simulink model "totalSystem"  (R2019b)
settings: Solver=FixedStepAuto  StartTime=0.0  StopTime=100.0  FixedStep=0.001  RelTol=1e-3
values from neighbouring files (symbols this model uses):
  ballLQRgain = lqr(ballSystem, Q, R)    [init.m]
  ballPosInit = [0.1;0;0;0]    [init.m]
  C_v = 16.5    [init.m]
  g = 9.81    [init.m]
  I0 = (m_p+3*m_m)*g/(3*K)    (= 0.37278)    [init.m]
  I_b = m_b*r_b^2    (= 8.664e-06)    [init.m]
  I_p = m_p*0.04^2/12    (= 0.00012)    [init.m]
  K = 11    [init.m]
  m_b = 0.024    [init.m]
  m_m = 0.118    [init.m]
  m_p = 0.9    [init.m]
  motorPlateInit = [0;0;0;0;0;0.32]    [init.m]
  r = 0.17    [init.m]
  r_b = 0.019    [init.m]
undefined symbols (not defined in the file or in its folder): Continuous, denc_mi, numc_mi, Time
libraries: ctrlSharedLib x1
settings Model: Creator=chukh  LastModifiedBy=chukh

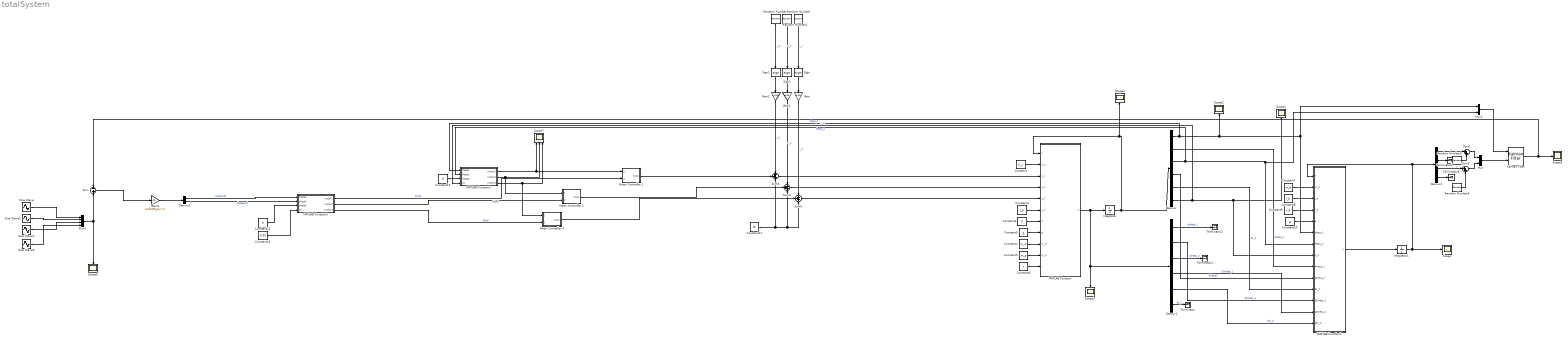
== system totalSystem ==
  Constant : Constant  Value=C_v
  Constant1 : Constant  Value=I_p
  Constant10 : Constant  Value=g
  Constant11 : Constant  Value=I0
  Constant12 : Constant  Value=0
  Constant13 : Constant  Value=0
  Constant14 : Constant  Value=0.32
  Constant2 : Constant  Value=K
  Constant3 : Constant  Value=g
  Constant4 : Constant  Value=m_m
  Constant5 : Constant  Value=m_p
  Constant6 : Constant  Value=r
  Constant7 : Constant  Value=m_b
  Constant8 : Constant  Value=I_b
  Constant9 : Constant  Value=r_b
  Demux : Demux  Outputs=6
  Demux1 : Demux  Outputs=6
  Demux2 : Demux
  Demux3 : Demux  Outputs=2
  Gain : Gain  Gain=0.05
  Gain1 : Gain  Gain=0.05
  Gain2 : Gain  Gain=0.05
  Gain3 : Gain  Gain=ballLQRgain  Multiplication=Matrix(K*u)
  Integrator : Integrator  InitialCondition=motorPlateInit
  Integrator1 : Integrator  InitialCondition=ballPosInit
  Kalman Filter : ctrlSharedLib/Kalman Filter  TimeDomain=Continuous-Time  UseCurrentEstimator=on  ModelSource=LTI State-Space Variable  ModelSourceVariable=ballSystem  A=0.95  B=1  C=1  D=0  NumberOfStates=1  NumberOfInputs=1  NumberOfOutputs=1  InitialEstimateSource=Dialog  X0=ballPosInit  P0=10  UseK=off  UseGH=off  NumberOfProcessNoiseInputs=1  G=1  TimeInvariantG=on  H=0  TimeInvariantH=on  Q=0.05  TimeInvariantQ=on  R=1  TimeInvariantR=on  N=0  TimeInvariantN=on  AddInputPort=on  AddEnablePort=off  OutputEstimatedY=off  OutputP=off  Ts=-1
      settings: SourceProductBaseCode=CT
  MATLAB Function : MATLAB Function  TreatAsAtomicUnit=on
  MATLAB Function1 : MATLAB Function  TreatAsAtomicUnit=on
  MATLAB Function2 : MATLAB Function  TreatAsAtomicUnit=on
  MATLAB Function3 : MATLAB Function  TreatAsAtomicUnit=on
  Motor Controller 1 : Subsystem
  Motor Controller 2 : Subsystem
  Motor Controller 3 : Subsystem
  Mux : Mux  Inputs=2
  Mux1 : Mux  Inputs=2
  Mux2 : Mux
  Random Number : RandomNumber  Seed=13  SampleTime=0.001
  Random Number1 : RandomNumber  Seed=23  SampleTime=0.001
  Random Number2 : RandomNumber  Seed=47  SampleTime=0.001
  Random Number3 : RandomNumber  Variance=0.005  Seed=193  SampleTime=0
  Random Number4 : RandomNumber  Variance=0.005  Seed=98676  SampleTime=0
  Scope{,1..6} (7 alike) : Scope
  Scope7 : Scope  NumInputPorts=3
  Sign : Signum
  Sign1 : Signum
  Sign2 : Signum
  Sine Wave : Sin  Amplitude=0.1  Frequency=pi/5  Phase=pi/2  SampleTime=0
  Sine Wave1 : Sin  Amplitude=0.1  Frequency=pi/5  SampleTime=0
  Sine Wave2 : Sin  Amplitude=0.1  Phase=pi  SampleTime=0
  Sine Wave3 : Sin  Amplitude=0.1  Phase=pi/2  SampleTime=0
  Sum : Sum  Inputs=-+
  Sum1 : Sum  Inputs=|++
  Sum2 : Sum  Inputs=|++
  Sum3 : Sum  Inputs=+++
  Sum4 : Sum  Inputs=+++
  Sum5 : Sum  Inputs=+++
  Terminator{,1..4} (5 alike) : Terminator
  wires:
  Demux/6 -> Scope1/1, MATLAB Function1/8(z_C), MATLAB Function2/4(Zc)  "z_C"
  Demux/2 -> MATLAB Function1/9(dtheta_1)  "dtheta_1"
  Demux/3 -> Mux1/2, MATLAB Function1/7(theta_2), MATLAB Function2/2(theta2)  "theta_2"
  Demux/4 -> MATLAB Function1/10(dtheta_2)  "dtheta2"
  Demux/5 -> MATLAB Function1/11(dz_C)  "dz_C"
  Demux1/6 -> Terminator/1  "dz_C"
  Demux1/1 -> Terminator2/1  "dtheta_1"
  Demux1/2 -> MATLAB Function1/12(d2theta_1)  "d2theta_1"
  Demux1/3 -> Terminator1/1  "dtheta_2"
  Demux1/4 -> MATLAB Function1/13(d2theta_2)  "d2theta_2"
  Demux1/5 -> MATLAB Function1/14(d2z_C)  "d2z_C"
  MATLAB Function1/1(V) -> Integrator1/1
  Integrator1/1 -> Scope/1, MATLAB Function1/1(Y), Demux2/1
  Constant7/1 -> MATLAB Function1/2(m_b)
  Constant8/1 -> MATLAB Function1/3(I_b)
  Constant9/1 -> MATLAB Function1/4(r_b)
  Constant10/1 -> MATLAB Function1/5(g)
  Demux/1 -> Scope2/1, MATLAB Function1/6(theta_1), Mux1/1, MATLAB Function2/1(theta1)  "theta_1"
  Constant5/1 -> MATLAB Function/10(m_p)
  MATLAB Function/1(V) -> Demux1/1, Scope3/1, Integrator/1
  Random Number/1 -> Sign/1  "I_1"
  Constant4/1 -> MATLAB Function/9(m_m)
  Integrator/1 -> Demux/1, Scope4/1, MATLAB Function/1(Y)
  Constant/1 -> MATLAB Function/2(C_v)
  Constant2/1 -> MATLAB Function/7(K)
  Random Number2/1 -> Sign2/1  "I_3"
  Constant6/1 -> MATLAB Function/11(r)
  Constant1/1 -> MATLAB Function/6(I_p)
  Random Number1/1 -> Sign1/1  "I_2"
  Constant3/1 -> MATLAB Function/8(g)
  Sign/1 -> Gain/1
  Sign1/1 -> Gain1/1
  Sign2/1 -> Gain2/1
  Sum3/1 -> MATLAB Function/4(I_2)
  Gain1/1 -> Sum3/1  "I_2"
  Gain2/1 -> Sum4/1  "I_1"
  Sum5/1 -> MATLAB Function/5(I_3)
  Constant11/1 -> Sum3/3, Sum5/3, Sum4/3
  Gain/1 -> Sum5/1  "I_3"
  Sum4/1 -> MATLAB Function/3(I_1)
  Constant12/1 -> MATLAB Function2/3(theta3)
  MATLAB Function2/1(motor1) -> Scope7/1, Motor Controller 1/1(Output)
  MATLAB Function3/1(motor1) -> Motor Controller 1/2(Reference)  "P1ref"
  Motor Controller 1/1(Out1) -> Sum4/2
  MATLAB Function3/2(motor2) -> Motor Controller 2/2(Reference)  "P2ref"
  MATLAB Function3/3(motor3) -> Motor Controller 3/2(Reference)  "P3ref"
  MATLAB Function2/2(motor2) -> Scope7/2, Motor Controller 2/1(Output)
  MATLAB Function2/3(motor3) -> Scope7/3, Motor Controller 3/1(Output)
  Motor Controller 3/1(Out1) -> Sum5/2
  Motor Controller 2/1(Out1) -> Sum3/2
  Demux2/2 -> Terminator3/1
  Demux2/4 -> Terminator4/1
  Demux2/1 -> Sum1/1  "x"
  Demux2/3 -> Sum2/1  "y"
  Mux/1 -> Kalman Filter/2
  Mux1/1 -> Kalman Filter/1
  Kalman Filter/1 -> Sum/1, Scope5/1
  Demux3/1 -> MATLAB Function3/1(theta1)  "theta1ref"
  Demux3/2 -> MATLAB Function3/2(theta2)  "theta2ref"
  Constant13/1 -> MATLAB Function3/3(theta3)
  Constant14/1 -> MATLAB Function3/4(Zc)
  Gain3/1 -> Demux3/1
  Sum/1 -> Gain3/1
  Sine Wave1/1 -> Mux2/3
  Mux2/1 -> Scope6/1, Sum/2
  Sine Wave2/1 -> Mux2/2
  Sine Wave/1 -> Mux2/1
  Sine Wave3/1 -> Mux2/4
  Random Number3/1 -> Sum1/2
  Random Number4/1 -> Sum2/2
  Sum2/1 -> Mux/2
  Sum1/1 -> Mux/1

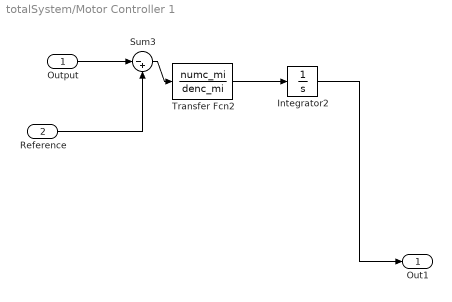
== system totalSystem/Motor Controller 1 ==
  Output : Inport
  Reference : Inport  Port=2
  Integrator2 : Integrator
  Sum3 : Sum  Inputs=|-+
  Transfer Fcn2 : TransferFcn  Numerator=numc_mi  Denominator=denc_mi
  Out1 : Outport
  wires:
  Transfer Fcn2/1 -> Integrator2/1
  Sum3/1 -> Transfer Fcn2/1
  Output/1 -> Sum3/1
  Reference/1 -> Sum3/2
  Integrator2/1 -> Out1/1

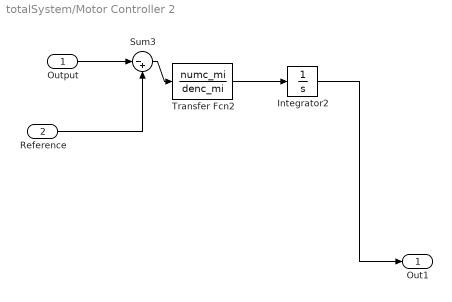
== system totalSystem/Motor Controller 2 ==
  Output : Inport
  Reference : Inport  Port=2
  Integrator2 : Integrator
  Sum3 : Sum  Inputs=|-+
  Transfer Fcn2 : TransferFcn  Numerator=numc_mi  Denominator=denc_mi
  Out1 : Outport
  wires:
  Transfer Fcn2/1 -> Integrator2/1
  Sum3/1 -> Transfer Fcn2/1
  Output/1 -> Sum3/1
  Reference/1 -> Sum3/2
  Integrator2/1 -> Out1/1

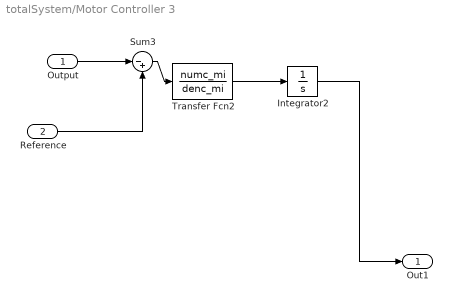
== system totalSystem/Motor Controller 3 ==
  Output : Inport
  Reference : Inport  Port=2
  Integrator2 : Integrator
  Sum3 : Sum  Inputs=|-+
  Transfer Fcn2 : TransferFcn  Numerator=numc_mi  Denominator=denc_mi
  Out1 : Outport
  wires:
  Transfer Fcn2/1 -> Integrator2/1
  Sum3/1 -> Transfer Fcn2/1
  Output/1 -> Sum3/1
  Reference/1 -> Sum3/2
  Integrator2/1 -> Out1/1

== matlab function totalSystem/MATLAB Function1 ==
  data: Y input; V output; m_b input; I_b input; r_b input; g input; theta_1 input; theta_2 input; z_C input; dtheta_1 input; dtheta_2 input; dz_C input; d2theta_1 input; d2theta_2 input; d2z_C input
function V = ballOnPlateODE(Y,m_b,I_b,r_b,g,theta_1,theta_2,z_C,dtheta_1,dtheta_2,dz_C,d2theta_1,d2theta_2,d2z_C)
%BALLONPLATEODE
%    V = BALLONPLATEODE(Y,M_B,I_B,R_B,G,THETA_1,THETA_2,Z_C,DTHETA_1,DTHETA_2,DZ_C,D2THETA_1,D2THETA_2,D2Z_C)

%    This function was generated by the Symbolic Math Toolbox version 8.4.
%    16-May-2021 00:03:52

%matrix([[xf], [Dxf], [yf], [Dyf]])
t2 = cos(theta_1);
t3 = cos(theta_2);
t4 = sin(theta_1);
t5 = sin(theta_2);
t6 = Y(1);
t7 = Y(2);
t8 = Y(3);
t9 = Y(4);
t10 = dtheta_1.^2;
t11 = dtheta_2.^2;
t12 = r_b.^2;
t13 = r_b.^3;
t14 = t2.^2;
t15 = t2.^3;
t16 = t3.^2;
t18 = t3.^3;
t20 = t4.^2;
t21 = t4.^3;
t22 = t5.^2;
t24 = t5.^3;
t28 = m_b.*t12;
t17 = t14.^2;
t19 = t16.^2;
t23 = t20.^2;
t25 = t22.^2;
t26 = 1.0./t14;
t27 = 1.0./t16;
t29 = I_b+t28;
t30 = t14+t20;
t31 = 1.0./t29;
t32 = 1.0./t30;
V = [t7;(t26.*t27.*t31.*t32.*(I_b.*d2theta_2.*r_b.*t15.*t18+I_b.*r_b.*t11.*t15.*t24.*2.0-I_b.*t6.*t11.*t17.*t19-I_b.*t6.*t11.*t17.*t25.*2.0+d2z_C.*t5.*t17.*t18.*t28+g.*t5.*t17.*t18.*t28+m_b.*t11.*t13.*t15.*t24.*2.0-t6.*t11.*t17.*t25.*t28.*2.0+d2theta_2.*m_b.*t3.*t13.*t15.*t22+d2theta_1.*t5.*t8.*t16.*t17.*t28-d2theta_2.*t5.*t6.*t17.*t18.*t28-d2theta_2.*t3.*t6.*t17.*t24.*t28+dtheta_1.*t5.*t9.*t16.*t17.*t28.*2.0-dtheta_2.*t5.*t7.*t17.*t18.*t28.*2.0+dtheta_1.*t5.*t9.*t17.*t18.*t28-dtheta_2.*t3.*t7.*t17.*t24.*t28.*2.0+m_b.*t5.*t10.*t13.*t15.*t16.*2.0+m_b.*t5.*t11.*t13.*t15.*t16+t4.*t8.*t11.*t15.*t24.*t28.*2.0-t6.*t10.*t16.*t17.*t22.*t28-t6.*t11.*t16.*t17.*t22.*t28.*2.0+I_b.*dtheta_1.*dtheta_2.*r_b.*t18.*t21.*2.0+I_b.*dtheta_1.*dtheta_2.*t8.*t17.*t18.*2.0-I_b.*dtheta_1.*dtheta_2.*t8.*t17.*t19+I_b.*dtheta_1.*dtheta_2.*t8.*t18.*t23.*2.0+I_b.*d2theta_2.*r_b.*t2.*t18.*t20+I_b.*d2theta_2.*r_b.*t3.*t15.*t22+I_b.*d2theta_1.*t5.*t8.*t16.*t17+I_b.*d2theta_2.*t4.*t8.*t15.*t18-I_b.*d2theta_2.*t5.*t6.*t17.*t18-I_b.*d2theta_1.*t5.*t8.*t17.*t18+I_b.*d2theta_2.*t2.*t8.*t18.*t21-I_b.*d2theta_2.*t3.*t6.*t17.*t24+I_b.*dtheta_1.*t5.*t9.*t16.*t17.*2.0+I_b.*dtheta_2.*t4.*t9.*t15.*t18.*2.0-I_b.*dtheta_2.*t5.*t7.*t17.*t18.*2.0-I_b.*dtheta_1.*t5.*t9.*t17.*t18+I_b.*dtheta_2.*t2.*t9.*t18.*t21.*2.0-I_b.*dtheta_2.*t3.*t7.*t17.*t24.*2.0+I_b.*r_b.*t5.*t10.*t15.*t16+I_b.*r_b.*t5.*t11.*t15.*t16.*2.0+I_b.*r_b.*t2.*t11.*t20.*t24.*2.0+I_b.*t4.*t8.*t11.*t15.*t24.*2.0+I_b.*t2.*t8.*t11.*t21.*t24.*2.0-I_b.*t6.*t11.*t14.*t19.*t20-I_b.*t6.*t11.*t16.*t17.*t22.*3.0-I_b.*t6.*t11.*t14.*t20.*t25.*2.0+I_b.*dtheta_1.*dtheta_2.*r_b.*t4.*t14.*t18.*2.0-I_b.*dtheta_1.*dtheta_2.*r_b.*t4.*t14.*t22+I_b.*dtheta_1.*dtheta_2.*r_b.*t3.*t21.*t22.*2.0+I_b.*dtheta_1.*dtheta_2.*t4.*t6.*t15.*t24+I_b.*dtheta_1.*dtheta_2.*t3.*t8.*t17.*t22.*2.0+I_b.*dtheta_1.*dtheta_2.*t3.*t8.*t22.*t23.*2.0+I_b.*dtheta_1.*dtheta_2.*t8.*t14.*t18.*t20.*4.0-I_b.*dtheta_1.*dtheta_2.*t8.*t14.*t19.*t20-I_b.*dtheta_1.*dtheta_2.*t8.*t14.*t20.*t22-I_b.*d2theta_1.*r_b.*t3.*t4.*t5.*t14+I_b.*d2theta_1.*r_b.*t4.*t5.*t14.*t16+I_b.*d2theta_2.*r_b.*t2.*t3.*t20.*t22+I_b.*d2theta_1.*t3.*t4.*t6.*t15.*t22-I_b.*d2theta_1.*t3.*t5.*t8.*t14.*t20+I_b.*d2theta_2.*t3.*t4.*t8.*t15.*t22+I_b.*d2theta_2.*t2.*t3.*t8.*t21.*t22+I_b.*d2theta_1.*t5.*t8.*t14.*t16.*t20-I_b.*d2theta_2.*t5.*t6.*t14.*t18.*t20-I_b.*d2theta_2.*t3.*t6.*t14.*t20.*t24+I_b.*dtheta_1.*t3.*t4.*t7.*t15.*t22-I_b.*dtheta_1.*t3.*t5.*t9.*t14.*t20+I_b.*dtheta_2.*t3.*t4.*t9.*t15.*t22.*2.0+I_b.*dtheta_2.*t2.*t3.*t9.*t21.*t22.*2.0+I_b.*dtheta_1.*t5.*t9.*t14.*t16.*t20.*2.0-I_b.*dtheta_2.*t5.*t7.*t14.*t18.*t20.*2.0-I_b.*dtheta_2.*t3.*t7.*t14.*t20.*t24.*2.0+I_b.*r_b.*t2.*t5.*t10.*t16.*t20+I_b.*r_b.*t2.*t5.*t11.*t16.*t20.*2.0-I_b.*t3.*t4.*t5.*t8.*t10.*t15+I_b.*t4.*t5.*t8.*t10.*t15.*t16+I_b.*t4.*t5.*t8.*t11.*t15.*t16.*2.0+I_b.*t4.*t5.*t8.*t10.*t15.*t18+I_b.*t2.*t5.*t8.*t10.*t16.*t21+I_b.*t2.*t5.*t8.*t11.*t16.*t21.*2.0-I_b.*t3.*t6.*t10.*t14.*t20.*t22-I_b.*t6.*t11.*t14.*t16.*t20.*t22.*3.0+dtheta_1.*dtheta_2.*m_b.*t4.*t13.*t14.*t22-dtheta_1.*dtheta_2.*t4.*t6.*t15.*t24.*t28+dtheta_1.*dtheta_2.*t3.*t8.*t17.*t22.*t28.*2.0+dtheta_1.*dtheta_2.*t8.*t14.*t20.*t22.*t28+d2theta_1.*m_b.*t4.*t5.*t13.*t14.*t16+d2theta_2.*t3.*t4.*t8.*t15.*t22.*t28+d2theta_1.*t5.*t8.*t14.*t16.*t20.*t28-dtheta_1.*t3.*t4.*t7.*t15.*t22.*t28+dtheta_1.*t3.*t5.*t9.*t14.*t20.*t28+dtheta_2.*t3.*t4.*t9.*t15.*t22.*t28.*2.0+dtheta_1.*t5.*t9.*t14.*t16.*t20.*t28.*2.0+m_b.*t2.*t3.*t5.*t10.*t13.*t20.*2.0+m_b.*t2.*t5.*t10.*t13.*t16.*t20+t3.*t4.*t5.*t8.*t10.*t15.*t28+t2.*t3.*t5.*t8.*t10.*t21.*t28.*2.0+t4.*t5.*t8.*t10.*t15.*t16.*t28+t4.*t5.*t8.*t11.*t15.*t16.*t28+t4.*t5.*t8.*t10.*t15.*t18.*t28+t2.*t5.*t8.*t10.*t16.*t21.*t28-t3.*t6.*t10.*t14.*t20.*t22.*t28+I_b.*dtheta_1.*dtheta_2.*r_b.*t3.*t4.*t14.*t22.*2.0+I_b.*dtheta_1.*dtheta_2.*t4.*t5.*t6.*t15.*t16+I_b.*dtheta_1.*dtheta_2.*t3.*t8.*t14.*t20.*t22.*4.0-I_b.*dtheta_1.*dtheta_2.*t8.*t14.*t16.*t20.*t22+dtheta_1.*dtheta_2.*m_b.*t3.*t4.*t13.*t14.*t22.*2.0+dtheta_1.*dtheta_2.*t3.*t8.*t14.*t20.*t22.*t28.*2.0))./(t16+t22);t9;-t26.*t27.*t31.*t32.*(I_b.*d2theta_1.*r_b.*t3.*t15+I_b.*r_b.*t10.*t16.*t21.*2.0+I_b.*t3.*t8.*t10.*t17+I_b.*t8.*t10.*t16.*t17-I_b.*t8.*t10.*t17.*t18+I_b.*t8.*t10.*t16.*t23.*2.0+d2z_C.*t4.*t15.*t18.*t28+g.*t4.*t15.*t18.*t28+m_b.*t10.*t13.*t16.*t21.*2.0-t3.*t8.*t10.*t17.*t28+t8.*t10.*t16.*t17.*t28.*2.0-t8.*t10.*t17.*t18.*t28+t8.*t10.*t16.*t23.*t28.*2.0+d2theta_1.*m_b.*t2.*t13.*t16.*t20+d2theta_1.*t4.*t8.*t15.*t16.*t28-d2theta_2.*t4.*t6.*t15.*t18.*t28+d2theta_1.*t2.*t8.*t16.*t21.*t28-dtheta_1.*t3.*t4.*t9.*t15.*t28+dtheta_1.*t3.*t5.*t7.*t17.*t28+dtheta_1.*t4.*t9.*t15.*t16.*t28.*2.0-dtheta_2.*t4.*t7.*t15.*t18.*t28.*2.0+dtheta_1.*t4.*t9.*t15.*t18.*t28+dtheta_1.*t2.*t9.*t16.*t21.*t28.*2.0-m_b.*t3.*t4.*t10.*t13.*t14.*2.0+m_b.*t4.*t10.*t13.*t14.*t16.*3.0+m_b.*t4.*t11.*t13.*t14.*t16+m_b.*t4.*t11.*t13.*t14.*t22.*2.0-t3.*t8.*t10.*t14.*t20.*t28.*2.0-t4.*t6.*t11.*t15.*t24.*t28.*2.0+t8.*t10.*t14.*t16.*t20.*t28.*4.0+t8.*t11.*t14.*t16.*t20.*t28+t8.*t11.*t14.*t20.*t22.*t28.*2.0+I_b.*dtheta_1.*dtheta_2.*r_b.*t5.*t15-I_b.*dtheta_1.*dtheta_2.*t6.*t16.*t17-I_b.*dtheta_1.*dtheta_2.*t6.*t17.*t22+I_b.*d2theta_1.*r_b.*t2.*t16.*t20+I_b.*d2theta_1.*t3.*t4.*t8.*t15-I_b.*d2theta_1.*t3.*t5.*t6.*t17+I_b.*d2theta_1.*t4.*t8.*t15.*t16-I_b.*d2theta_1.*t4.*t8.*t15.*t18+I_b.*d2theta_1.*t2.*t8.*t16.*t21+I_b.*dtheta_1.*t3.*t4.*t9.*t15-I_b.*dtheta_1.*t3.*t5.*t7.*t17+I_b.*dtheta_1.*t4.*t9.*t15.*t16.*2.0-I_b.*dtheta_1.*t4.*t9.*t15.*t18+I_b.*dtheta_1.*t2.*t9.*t16.*t21.*2.0+I_b.*r_b.*t4.*t10.*t14.*t16.*2.0+I_b.*t8.*t10.*t14.*t16.*t20.*3.0-dtheta_1.*dtheta_2.*m_b.*t5.*t13.*t15+dtheta_1.*dtheta_2.*t6.*t17.*t22.*t28+I_b.*dtheta_1.*dtheta_2.*t4.*t5.*t8.*t15+I_b.*t3.*t4.*t5.*t6.*t10.*t15-dtheta_1.*dtheta_2.*t4.*t5.*t8.*t15.*t28+d2theta_2.*m_b.*t3.*t4.*t5.*t13.*t14-d2theta_2.*t3.*t4.*t6.*t15.*t22.*t28+d2theta_2.*t3.*t5.*t8.*t14.*t20.*t28-dtheta_2.*t3.*t4.*t7.*t15.*t22.*t28.*2.0+dtheta_2.*t3.*t5.*t9.*t14.*t20.*t28.*2.0+t3.*t4.*t5.*t6.*t10.*t15.*t28-t4.*t5.*t6.*t10.*t15.*t16.*t28-t4.*t5.*t6.*t11.*t15.*t16.*t28.*2.0+I_b.*dtheta_1.*dtheta_2.*t4.*t5.*t8.*t15.*t16+dtheta_1.*dtheta_2.*m_b.*t2.*t3.*t5.*t13.*t20.*2.0+dtheta_1.*dtheta_2.*t3.*t4.*t5.*t8.*t15.*t28.*2.0+dtheta_1.*dtheta_2.*t2.*t3.*t5.*t8.*t21.*t28.*2.0)];

== matlab function totalSystem/MATLAB Function ==
  data: V output; Y input; C_v input; I_1 input; I_2 input; I_3 input; I_p input; K input; g input; m_m input; m_p input; r input
function V = motorPlateODE(Y,C_v,I_1,I_2,I_3,I_p,K,g,m_m,m_p,r)
%MOTORPLATEODE
%    V = MOTORPLATEODE(T,Y,C_V,I_1,I_2,I_3,I_P,K,G,M_M,M_P,R)

%    This function was generated by the Symbolic Math Toolbox version 8.4.
%    18-May-2021 19:45:09

%matrix([[theta_1f], [omega_1f], [theta_2f], [omega_2f], [dz_Cf], [z_Cf]])
t2 = I_p.^2;
t3 = Y(1);
t4 = Y(2);
t5 = Y(3);
t6 = Y(4);
t7 = Y(5);
t8 = m_m.^2;
t9 = r.^2;
t10 = r.^3;
t19 = sqrt(3.0);
t11 = t9.^2;
t12 = cos(t3);
t13 = cos(t5);
t14 = sin(t3);
t15 = sin(t5);
t16 = t2.*4.0;
t17 = t4.^2;
t18 = t6.^2;
t20 = t12.^2;
t21 = t12.^3;
t22 = t13.^2;
t23 = t13.^3;
t25 = t14.^2;
t26 = t15.^2;
t24 = t22.^2;
t27 = I_p.*m_m.*t9.*t22.*6.0;
t29 = I_p.*m_m.*t9.*t25.*t26.*6.0;
t28 = t20.*t27;
t30 = t8.*t11.*t20.*t24.*9.0;
t31 = t16+t27+t28+t29+t30;
t32 = 1.0./t31;
V = [t4;t32.*(t12.*t14.*t17.*t27+t12.*t14.*t18.*t27+t8.*t11.*t12.*t14.*t17.*t24.*9.0+t8.*t11.*t12.*t14.*t18.*t24.*9.0-C_v.*I_p.*t4.*t9.*t20.*t22.*6.0-C_v.*m_m.*t4.*t11.*t20.*t24.*9.0+I_2.*I_p.*K.*r.*t12.*t13.*t19.*2.0-I_3.*I_p.*K.*r.*t12.*t13.*t19.*2.0+I_2.*K.*m_m.*t10.*t12.*t19.*t23.*3.0-I_3.*K.*m_m.*t10.*t12.*t19.*t23.*3.0+t4.*t6.*t8.*t11.*t15.*t20.*t23.*1.8e+1+t8.*t11.*t12.*t14.*t18.*t22.*t26.*1.8e+1-t8.*t11.*t14.*t18.*t21.*t22.*t26.*9.0-t8.*t11.*t12.*t14.^3.*t18.*t22.*t26.*9.0-t4.*t6.*t8.*t11.*t13.*t15.^3.*t20.*t25.*9.0+C_v.*I_p.*t6.*t9.*t12.*t13.*t14.*t15.*6.0-I_1.*K.*m_m.*t10.*t12.*t14.*t15.*t22.*6.0+I_2.*K.*m_m.*t10.*t12.*t14.*t15.*t22.*3.0+I_3.*K.*m_m.*t10.*t12.*t14.*t15.*t22.*3.0+I_p.*m_m.*t4.*t6.*t9.*t13.*t15.*t20.*1.2e+1+t4.*t6.*t8.*t11.*t13.*t15.*t20.*t25.*9.0-t4.*t6.*t8.*t11.*t15.*t20.*t23.*t25.*9.0);t6;-r.*t32.*(I_1.*I_p.*K.*t13.*4.0-I_2.*I_p.*K.*t13.*2.0-I_3.*I_p.*K.*t13.*2.0+C_v.*I_p.*r.*t6.*t22.*6.0-t8.*t10.*t15.*t18.*t20.*t23.*1.8e+1+t8.*t10.*t15.*t18.*t20.^2.*t23.*9.0+I_2.*I_p.*K.*t14.*t15.*t19.*2.0-I_3.*I_p.*K.*t14.*t15.*t19.*2.0+C_v.*I_p.*r.*t6.*t25.*t26.*6.0+I_1.*K.*m_m.*t9.*t20.*t23.*6.0-I_2.*K.*m_m.*t9.*t20.*t23.*3.0-I_3.*K.*m_m.*t9.*t20.*t23.*3.0+C_v.*m_m.*t6.*t10.*t20.*t24.*9.0-I_p.*m_m.*r.*t13.*t15.*t18.*1.2e+1-I_p.*m_m.*r.*t4.*t6.*t12.*t14.*6.0+I_p.*m_m.*r.*t13.*t15.*t18.*t20.*6.0+I_p.*m_m.*r.*t13.*t15.*t17.*t25.*6.0+I_p.*m_m.*r.*t13.*t15.*t18.*t25.*1.2e+1-t4.*t6.*t8.*t10.*t14.*t21.*t22.*9.0+t4.*t6.*t8.*t10.*t14.*t21.*t24.*9.0+t8.*t10.*t15.*t18.*t20.*t23.*t25.*9.0-C_v.*I_p.*r.*t4.*t12.*t13.*t14.*t15.*6.0+I_p.*m_m.*r.*t4.*t6.*t12.*t14.*t22.*6.0+I_p.*m_m.*r.*t4.*t6.*t12.*t14.*t26.*1.8e+1+t4.*t6.*t8.*t10.*t14.*t21.*t22.*t26.*9.0);-(C_v.*t7.*3.0+g.*m_m.*3.0+g.*m_p-I_1.*K-I_2.*K-I_3.*K)./(m_m.*3.0+m_p);t7];

== matlab function totalSystem/MATLAB Function2 ==
  data: theta1 input; motor1 output; theta2 input; theta3 input; Zc input; motor2 output; motor3 output
% Roll-Pitch-Yaw angles to motors position
% Roll (theta1): rotation about x-axis
% Pitch (theta2): rotation about y-axis
% Yaw (theta3): rotation about z-axis
% See page 12 and Appendix A (Multibody and Nonlinear Dynamics lecture
% notes for further reference
% Motors (1,2,3) -> (A,B,C)

function [motor1, motor2, motor3] = anglesToMotors(theta1,theta2,theta3,Zc)

%% Define parameters
r = 0.17;
r0B1 = [r; 0; 0];      
r0B2 = [-0.5*r; (sqrt(3)/2)*r; 0];
r0B3 = [-0.5*r; -(sqrt(3)/2)*r; 0];
r0B = [r0B1 r0B2 r0B3];
%r1C1 = r0B1; r1C2 = r0B2; r1C3 = r0B3;
r1C = r0B;
r0Oc = [0;0;Zc];

% Find cos and sin to accelerate calculations
C1 = cos(theta1);S1 = sin(theta1);C2 = cos(theta2);S2 = sin(theta2);C3 = cos(theta3);S3 = sin(theta3);

% Rotation matrices
RotZ = [C3 S3 0; -S3 C3 0; 0 0 1];
RotY = [C2 0 -S2; 0 1 0; S2 0 C2];
RotX = [1 0 0; 0 C1 S1; 0 -S1 C1];

A10 = RotX*RotY*RotZ; A01 = A10';

% Find rCiBi (Vectors representing the motors)
rCiBi = zeros(3,3);
for i=1:3
    rCiBi(:,i) = r0Oc + A01*r1C(:,i) - r0B(:,i);
end

% Outputs to motor are the lengths of the vectors
motor1 = norm(rCiBi(:,1));
motor2 = norm(rCiBi(:,2));
motor3 = norm(rCiBi(:,3));
end

== matlab function totalSystem/MATLAB Function3 ==
  data: theta1 input; motor1 output; theta2 input; theta3 input; Zc input; motor2 output; motor3 output
% Roll-Pitch-Yaw angles to motors position
% Roll (theta1): rotation about x-axis
% Pitch (theta2): rotation about y-axis
% Yaw (theta3): rotation about z-axis
% See page 12 and Appendix A (Multibody and Nonlinear Dynamics lecture
% notes for further reference
% Motors (1,2,3) -> (A,B,C)

function [motor1, motor2, motor3] = anglesToMotors(theta1,theta2,theta3,Zc)

%% Define parameters
r = 0.17;
r0B1 = [r; 0; 0];      
r0B2 = [-0.5*r; (sqrt(3)/2)*r; 0];
r0B3 = [-0.5*r; -(sqrt(3)/2)*r; 0];
r0B = [r0B1 r0B2 r0B3];
%r1C1 = r0B1; r1C2 = r0B2; r1C3 = r0B3;
r1C = r0B;
r0Oc = [0;0;Zc];

% Find cos and sin to accelerate calculations
C1 = cos(theta1);S1 = sin(theta1);C2 = cos(theta2);S2 = sin(theta2);C3 = cos(theta3);S3 = sin(theta3);

% Rotation matrices
RotZ = [C3 S3 0; -S3 C3 0; 0 0 1];
RotY = [C2 0 -S2; 0 1 0; S2 0 C2];
RotX = [1 0 0; 0 C1 S1; 0 -S1 C1];

A10 = RotX*RotY*RotZ; A01 = A10';

% Find rCiBi (Vectors representing the motors)
rCiBi = zeros(3,3);
for i=1:3
    rCiBi(:,i) = r0Oc + A01*r1C(:,i) - r0B(:,i);
end

% Outputs to motor are the lengths of the vectors
motor1 = norm(rCiBi(:,1));
motor2 = norm(rCiBi(:,2));
motor3 = norm(rCiBi(:,3));
end
